simulink model "Sim_3_observer_performance_no_noise"  (R2019b)
settings: Solver=VariableStepAuto  StartTime=0.0  StopTime=sim_time  FixedStep=0.01  MaxStep=0.1  MinStep=0.0001  RelTol=0.01  AbsTol=0.01
values from neighbouring files (symbols this model uses):
  Controller_Data = struct('K_p', K_p, 'K_v', K_v, 'K_i', K_i, 'M', M,     'D', D, 'U_ref', U_ref, 'mu', mu)    [Sim_10_init.m]    (also in Sim_11_init.m; Sim_12_init.m; Sim_3_4_and_5_init.m; Sim_7_8_userdef_init.m)
  D = [ 0.66  0    0 ... (first row only)    [Sim_10_init.m]    (also in Sim_11_init.m; Sim_12_init.m; Sim_3_4_and_5_init.m; Sim_7_8_userdef_init.m)
  K_p = 0.08*[1.1  0    0 ... (first row only)    [Sim_10_init.m]    (also in Sim_11_init.m; Sim_12_init.m; Sim_3_4_and_5_init.m; Sim_7_8_userdef_init.m)
  K_v = 1*[10   0       0 ... (first row only)    [Sim_10_init.m]    (also in Sim_11_init.m; Sim_12_init.m; Sim_3_4_and_5_init.m; Sim_7_8_userdef_init.m = 3*[10   0       0)
  LossOfSignalFalse = 1    [Sim_10_init.m]    (also in Sim_11_init.m; Sim_12_init.m; Sim_3_4_and_5_init.m; Sim_7_8_userdef_init.m)
  LossOfSignalTime = 10    [Sim_10_init.m]    (also in Sim_11_init.m; Sim_12_init.m; Sim_3_4_and_5_init.m = 30; Sim_7_8_userdef_init.m)
  LossOfSignalTrue = 0    [Sim_10_init.m]    (also in Sim_11_init.m; Sim_12_init.m; Sim_3_4_and_5_init.m; Sim_7_8_userdef_init.m)
  M = [ 16    0      0 ... (first row only)    [Sim_10_init.m]    (also in Sim_11_init.m; Sim_12_init.m; Sim_3_4_and_5_init.m; Sim_7_8_userdef_init.m)
  mu = 0.09    [Sim_10_init.m]    (also in Sim_11_init.m; Sim_12_init.m; Sim_3_4_and_5_init.m; Sim_7_8_userdef_init.m)
  Observergains = [L1, L2, L3]    [Sim_10_init.m]    (also in Sim_11_init.m; Sim_12_init.m; Sim_3_4_and_5_init.m; Sim_7_8_userdef_init.m)
  path_planner_data = [start_pos; end_pos; Radius; Center]    [Sim_10_init.m]    (also in Sim_11_init.m; Sim_12_init.m; Sim_3_4_and_5_init.m; Sim_7_8_userdef_init.m)
  pathparameter = 0    [Sim_10_init.m]    (also in Sim_11_init.m = 1; Sim_12_init.m; Sim_3_4_and_5_init.m = 1; Sim_7_8_userdef_init.m = 1)
  RegainOfSignalFalse = 0    [Sim_10_init.m]    (also in Sim_11_init.m; Sim_12_init.m; Sim_3_4_and_5_init.m; Sim_7_8_userdef_init.m)
  RegainOfSignalTime = 30    [Sim_10_init.m]    (also in Sim_11_init.m; Sim_12_init.m; Sim_3_4_and_5_init.m = 50; Sim_7_8_userdef_init.m)
  RegainOfSignalTrue = 1    [Sim_10_init.m]    (also in Sim_11_init.m; Sim_12_init.m; Sim_3_4_and_5_init.m; Sim_7_8_userdef_init.m)
  start_pos = [10; 20; pi/2 ]    [Sim_10_init.m]    (also in Sim_11_init.m = [0; 0; 0 ]; Sim_12_init.m = [0; 0; 0 ]; Sim_3_4_and_5_init.m = [0; 0; 0 ]; Sim_7_init.m = [0; 0; 0 ])
undefined symbols (not defined in the file or in its folder): tsamp, WP
(part 2 of 3)

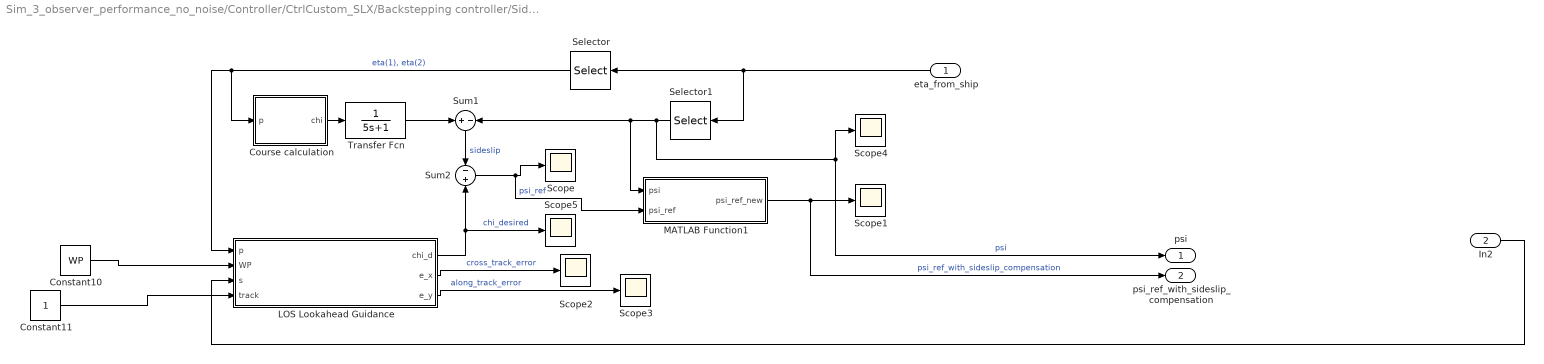
== system Sim_3_observer_performance_no_noise/Controller/CtrlCustom_SLX/Backstepping controller/Sideslip compensation  ==
  eta_from_ship : Inport
  In2 : Inport  Port=2
  Constant10 : Constant  Value=WP
  Constant11 : Constant
  Course calculation : MATLAB Function  TreatAsAtomicUnit=on  SystemSampleTime=tsamp
  LOS Lookahead Guidance : MATLAB Function  TreatAsAtomicUnit=on  SystemSampleTime=tsamp
  MATLAB Function1 : MATLAB Function  TreatAsAtomicUnit=on
  Scope{,1..5} (6 alike) : Scope
  Selector : Selector  InputPortWidth=3  IndexOptions=Index vector (dialog)  Indices=[1 2]  OutputSizes=1
  Selector1 : Selector  InputPortWidth=3  IndexOptions=Index vector (dialog)  Indices=[3]  OutputSizes=1
  Sum1 : Sum  Inputs=+-
  Sum2 : Sum  Inputs=-+
  Transfer Fcn : TransferFcn  Denominator=[5 1]
  psi : Outport
  psi_ref_with_sideslip_compensation : Outport  Port=2
  wires:
  Constant11/1 -> LOS Lookahead Guidance/4(track)
  Selector/1 -> LOS Lookahead Guidance/1(p), Course calculation/1(p)  "eta(1), eta(2)"
  eta_from_ship/1 -> Selector1/1, Selector/1
  Course calculation/1(chi) -> Transfer Fcn/1
  Sum1/1 -> Sum2/1  "sideslip"
  LOS Lookahead Guidance/1(chi_d) -> Sum2/2, Scope5/1  "chi_desired"
  Sum2/1 -> MATLAB Function1/2(psi_ref), Scope/1  "psi_ref"
  Transfer Fcn/1 -> Sum1/1
  LOS Lookahead Guidance/3(e_y) -> Scope3/1  "along_track_error"
  Selector1/1 -> psi/1, Scope4/1, Sum1/2, MATLAB Function1/1(psi)  "psi"
  In2/1 -> LOS Lookahead Guidance/3(s)
  Constant10/1 -> LOS Lookahead Guidance/2(WP)
  LOS Lookahead Guidance/2(e_x) -> Scope2/1  "cross_track_error"
  MATLAB Function1/1(psi_ref_new) -> psi_ref_with_sideslip_compensation/1, Scope1/1  "psi_ref_with_sideslip_compensation"

== system Sim_3_observer_performance_no_noise/Controller/DP_Ctrl/Backstepping controller/1//|p_d'| ==
  s : Inport
  switch : Inport  Port=2
  Elipse : MATLAB Function  TreatAsAtomicUnit=on
  Straight line : MATLAB Function  TreatAsAtomicUnit=on
  Switch : Switch  Criteria=u2 > Threshold
  1/|p_d'| : Outport
  wires:
  s/1 -> Elipse/1(s)
  Elipse/1(y) -> Switch/3
  Switch/1 -> 1/|p_d'|/1
  Straight line/1(y) -> Switch/1
  switch/1 -> Switch/2

== system Sim_3_observer_performance_no_noise/Controller/DP_Ctrl/Backstepping controller/Final_Tau_Computation ==
  alpha_1 : Inport
  alpha_1_dot : Inport  Port=2
  nu_hat : Inport  Port=3
  Gain : Gain  Gain=K_v  Multiplication=Matrix(K*u)
  Gain1 : Gain  Gain=M  Multiplication=Matrix(K*u)
  Gain2 : Gain  Gain=D  Multiplication=Matrix(K*u)
  Sum : Sum  Inputs=-+|
  Sum1 : Sum  Inputs=++-
  Tau : Outport
  wires:
  nu_hat/1 -> Sum/2
  alpha_1/1 -> Gain2/1, Sum/1
  Sum/1 -> Gain/1  "z_2"
  Sum1/1 -> Tau/1
  Gain/1 -> Sum1/3
  alpha_1_dot/1 -> Gain1/1
  Gain1/1 -> Sum1/1
  Gain2/1 -> Sum1/2

== system Sim_3_observer_performance_no_noise/Controller/DP_Ctrl/Backstepping controller/U_s(s) ==
  s : Inport
  switch : Inport  Port=2
  Eliptical : MATLAB Function  TreatAsAtomicUnit=on
  Straight line : MATLAB Function  TreatAsAtomicUnit=on
  Switch : Switch  Criteria=u2 > Threshold
  U_s : Outport
  wires:
  Straight line/1(y) -> Switch/1
  Switch/1 -> U_s/1
  Eliptical/1(y) -> Switch/3
  s/1 -> Eliptical/1(s)
  switch/1 -> Switch/2

== system Sim_3_observer_performance_no_noise/Controller/DP_Ctrl/Backstepping controller/U_s(s)' ==
  s : Inport
  "switch " : Inport  Port=2
  Constant : Constant  Value=0
  Elliptical : MATLAB Function  TreatAsAtomicUnit=on
  Switch : Switch  Criteria=u2 > Threshold
  U_s' : Outport
  wires:
  s/1 -> Elliptical/1(s)
  Elliptical/1(U_sf) -> Switch/3
  Switch/1 -> U_s'/1
  Constant/1 -> Switch/1
  "switch "/1 -> Switch/2

== system Sim_3_observer_performance_no_noise/Controller/DP_Ctrl/Backstepping controller/alpha_1, z_1 - explicit  ==
  eta : Inport
  eta_d(s) : Inport  Port=2
  eta_d(s)' : Inport  Port=3
  U_s : Inport  Port=4
  Gain : Gain  Gain=-K_p
  Product : Product
  Product1 : Product  Inputs=3
  Rotation Matrix : MATLAB Function  TreatAsAtomicUnit=on
  Selector : Selector  InputPortWidth=3  IndexOptions=Index vector (dialog)  Indices=[3]  OutputSizes=1
  Sum : Sum  Inputs=|+-
  Sum1 : Sum  Inputs=|++
  Transpose : Math  Operator=transpose  SignedPower=off  SaturateOnIntegerOverflow=on
  alpha_1 : Outport
  z_1 : Outport  Port=2
  wires:
  eta/1 -> Sum/1, Selector/1
  Selector/1 -> Rotation Matrix/1(psi)
  eta_d(s)/1 -> Sum/2
  Sum/1 -> Product/2
  Rotation Matrix/1(R_psi) -> Transpose/1
  Product/1 -> Gain/1, z_1/1
  Gain/1 -> Sum1/1
  Sum1/1 -> alpha_1/1
  Transpose/1 -> Product1/1, Product/1
  Product1/1 -> Sum1/2
  eta_d(s)'/1 -> Product1/2
  U_s/1 -> Product1/3

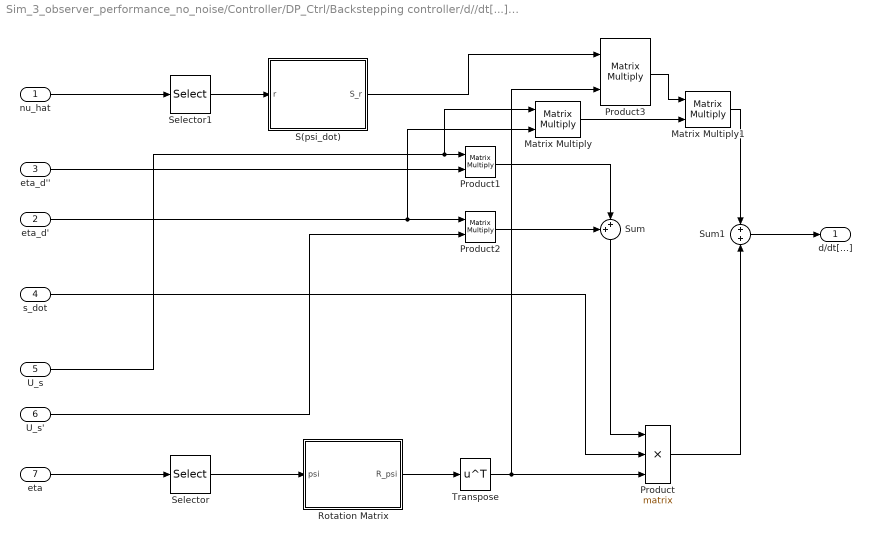
== system Sim_3_observer_performance_no_noise/Controller/DP_Ctrl/Backstepping controller/d//dt[...] calculation subsystem ==
  nu_hat : Inport
  eta_d' : Inport  Port=2
  eta_d'' : Inport  Port=3
  s_dot : Inport  Port=4
  U_s : Inport  Port=5
  "U_s' " : Inport  Port=6
  "eta " : Inport  Port=7
  Matrix Multiply : Product  Multiplication=Matrix(*)
  Matrix Multiply1 : Product  Multiplication=Matrix(*)
  Product : Product  Inputs=3  Multiplication=Matrix(*)
  Product1 : Product  Multiplication=Matrix(*)
  Product2 : Product  Multiplication=Matrix(*)
  Product3 : Product  Multiplication=Matrix(*)
  Rotation Matrix : MATLAB Function  TreatAsAtomicUnit=on
  S(psi_dot) : MATLAB Function  TreatAsAtomicUnit=on
  Selector : Selector  InputPortWidth=3  IndexOptions=Index vector (dialog)  Indices=[3]  OutputSizes=1
  Selector1 : Selector  InputPortWidth=3  IndexOptions=Index vector (dialog)  Indices=[3]  OutputSizes=1
  Sum : Sum  Inputs=++|
  Sum1 : Sum
  Transpose : Math  Operator=transpose  SignedPower=off  SaturateOnIntegerOverflow=on
  d/dt[...] : Outport
  wires:
  "eta "/1 -> Selector/1
  Selector/1 -> Rotation Matrix/1(psi)
  Rotation Matrix/1(R_psi) -> Transpose/1
  Transpose/1 -> Product3/2, Product/3
  s_dot/1 -> Product/2
  eta_d''/1 -> Product1/2
  U_s/1 -> Matrix Multiply/1, Product1/1
  Sum/1 -> Product/1
  Product1/1 -> Sum/2
  eta_d'/1 -> Matrix Multiply/2, Product2/1
  "U_s' "/1 -> Product2/2
  Product2/1 -> Sum/1
  nu_hat/1 -> Selector1/1
  Selector1/1 -> S(psi_dot)/1("r ")
  S(psi_dot)/1(S_r) -> Product3/1
  Product/1 -> Sum1/2
  Sum1/1 -> d/dt[...]/1
  Matrix Multiply/1 -> Matrix Multiply1/2
  Product3/1 -> Matrix Multiply1/1
  Matrix Multiply1/1 -> Sum1/1

== system Sim_3_observer_performance_no_noise/Controller/DP_Ctrl/Backstepping controller/eta_d''(s) ==
  s : Inport
  switch : Inport  Port=2
  Constant : Constant  Value=[0 0 0]'
  Elliptical : MATLAB Function  TreatAsAtomicUnit=on
  Switch : Switch  Criteria=u2 > Threshold
  "eta_d''(s) " : Outport
  wires:
  s/1 -> Elliptical/1(s)
  Elliptical/1(y) -> Switch/3
  Switch/1 -> "eta_d''(s) "/1
  Constant/1 -> Switch/1
  switch/1 -> Switch/2

== system Sim_3_observer_performance_no_noise/Controller/DP_Ctrl/Backstepping controller/eta_d'(s) ==
  s : Inport
  switch : Inport  Port=2
  Elliptical : MATLAB Function  TreatAsAtomicUnit=on
  Straight line : MATLAB Function  TreatAsAtomicUnit=on
  Switch : Switch  Criteria=u2 > Threshold
  Out1 : Outport
  wires:
  s/1 -> Elliptical/1(s)
  Elliptical/1(y) -> Switch/3
  Switch/1 -> Out1/1
  Straight line/1(y) -> Switch/1
  switch/1 -> Switch/2

== system Sim_3_observer_performance_no_noise/Controller/DP_Ctrl/Backstepping controller/eta_d(s) ==
  s : Inport
  switch : Inport  Port=2
  Eliptical path : MATLAB Function  TreatAsAtomicUnit=on
  Straight line : MATLAB Function  TreatAsAtomicUnit=on
  Switch : Switch  Criteria=u2 > Threshold
  "eta_d''(s) " : Outport
  wires:
  s/1 -> Straight line/1(s), Eliptical path/1(s)
  Eliptical path/1(y) -> Switch/3
  Switch/1 -> "eta_d''(s) "/1
  Straight line/1(y) -> Switch/1
  switch/1 -> Switch/2

== system Sim_3_observer_performance_no_noise/Controller/DP_Ctrl/Backstepping controller/z_1_dot subsystem  ==
  eta_d : Inport
  eta_d' : Inport  Port=2
  eta : Inport  Port=3
  s_dot : Inport  Port=4
  nu_hat : Inport  Port=5
  Product : Product  Inputs=3  Multiplication=Matrix(*)
  Product1 : Product  Inputs=3  Multiplication=Matrix(*)
  Rotation Matrix : MATLAB Function  TreatAsAtomicUnit=on
  S(psi_dot) : MATLAB Function  TreatAsAtomicUnit=on
  Selector : Selector  InputPortWidth=3  IndexOptions=Index vector (dialog)  Indices=[3]  OutputSizes=1
  Selector1 : Selector  InputPortWidth=3  IndexOptions=Index vector (dialog)  Indices=[3]  OutputSizes=1
  Sum : Sum  Inputs=-+|
  Sum1 : Sum  Inputs=+++
  Transpose : Math  Operator=transpose  SignedPower=off  SaturateOnIntegerOverflow=on
  Transpose1 : Math  Operator=transpose  SignedPower=off  SaturateOnIntegerOverflow=on
  Transpose3 : Math  Operator=transpose  SignedPower=off  SaturateOnIntegerOverflow=on
  z_1_dot : Outport
  wires:
  nu_hat/1 -> Sum1/3, Selector/1
  Selector/1 -> S(psi_dot)/1("r ")
  eta/1 -> Selector1/1, Sum/2
  eta_d/1 -> Sum/1
  Selector1/1 -> Rotation Matrix/1(psi)
  Rotation Matrix/1(R_psi) -> Transpose1/1
  Sum/1 -> Product/1
  S(psi_dot)/1(S_r) -> Transpose/1
  Transpose/1 -> Product/3
  Sum1/1 -> Transpose3/1
  Product/1 -> Sum1/2
  s_dot/1 -> Product1/2
  eta_d'/1 -> Product1/1
  Product1/1 -> Sum1/1
  Transpose1/1 -> Product/2, Product1/3
  Transpose3/1 -> z_1_dot/1

== system Sim_3_observer_performance_no_noise/Controller/DP_Ctrl/Thrust Allocation /u ==
  In1 : Inport
  Constant : Constant  Value=0.3
  Constant1 : Constant  Value=0.3
  Demux1 : Demux  Outputs=5
  Mux : Mux  Inputs=7
  Saturation1 : Saturate  UpperLimit=1  LowerLimit=0
  Saturation11 : Saturate  UpperLimit=1  LowerLimit=0
  Out1 : Outport  VectorParamsAs1DForOutWhenUnconnected=off
  wires:
  In1/1 -> Demux1/1
  Demux1/1 -> Mux/1  "u_BT"
  Demux1/2 -> Saturation11/1  "u_VSP1"
  Demux1/3 -> Saturation1/1  "u_VSP2"
  Demux1/4 -> Mux/4  "alpha_VSP1"
  Demux1/5 -> Mux/5  "alpha_VSP2"
  Constant/1 -> Mux/6  "omega_VSP1"
  Constant1/1 -> Mux/7  "omega_VSP2"
  Mux/1 -> Out1/1
  Saturation11/1 -> Mux/2
  Saturation1/1 -> Mux/3

== matlab function Sim_3_observer_performance_no_noise/Simulator CSE1/EquationsOfMotion (Fossen Model)/kinematics ==
  data: nu input size=3; eta_dot output size=3; eta input size=3
function eta_dot = CSE1_eta_dot(nu,eta)

psi = eta(3);

J = [cos(psi) -sin(psi) 0
     sin(psi) cos(psi)  0
     0        0         1];

eta_dot = J*nu;

== matlab function Sim_3_observer_performance_no_noise/Simulator CSE1/EquationsOfMotion (Fossen Model)/kinetics ==
  data: tau input; nu_dot output; nu input
function nu_dot = CSE1_nu_dot(tau,nu)

u   = nu(1);
v   = nu(2);
r   = nu(3);

tau = [tau(1);tau(2);tau(3)];
%% MATRICES 
%changed m from 14.79 to 14.11

m    = 14.11;   I_z  =  1.7600;   x_g = 0.0375;       % x_g  =  0.0460; % Table B.1

%% Added mass
%changed Y_vd from -1.0 to -10.0
X_ud  =     -2.0;											% Table B.1
					Y_vd =      -10.0;	N_vd =    -0.0;		% Table B.1
					Y_rd =      -0.0;	N_rd =    -1.0;		% Table B.1

%% Total mass matrix
m_11 = m-X_ud;
m_22 = m-Y_vd;
m_23 = m*x_g-Y_rd;
m_32 = m*x_g-N_vd; % noted as Y_rd in handbook, but same value
m_33 = I_z-N_rd;

M    = [m_11 0    0
        0    m_22 m_23
        0    m_32 m_33];
	
%% Damping coefficients
% Comments at the end of the lines indicate the old values used.
X_u		= -0.6555;		X_v		= 0;
X_uu 	= 0.3545;		X_vv	= -2.443;
X_uuu 	= -3.787;		X_vvv	= 0;

						Y_v		= -1.33; 			Y_r		= -7.250; % Y_r
						Y_vv	= -2.776;			Y_rr	= -3.450; % Y_rr
						Y_vvv	= -64.91;			Y_rrr	= 0;
						
						Y_rv	= -0.805;			Y_vr	= -0.845; % Y_rv, Y_vr

						N_v		= 0;				N_r		= -1.900; % N_r
						N_vv	= -0.2088;			N_rr	= -0.750; % N_rr
						N_vvv	= 0;				N_rrr	= 0;
						
						N_rv	= 0.130;			N_vr	= 0.080; % N_rv, N_vr

%% Correolis matrix
c_13 = -(m-Y_vd)*v-(m*x_g-Y_rd)*r;
c_23 = (m-X_ud)*u;
C    = [0     0     c_13
        0     0     c_23
        -c_13 -c_23 0   ];

%% Assembly of the damping matrix
%should be abs(u), abs(v) some places, only positive values? 

d_11 = -X_u - X_uu*u - X_uuu*u^2;
d_22 = -Y_v - Y_vv*v - Y_vvv*v^2 - Y_rv*abs(r);
d_33 = -N_r - N_rr*abs(r) - N_rrr*r^2 - N_vr*abs(v); % using abs(r)

d_12 = -X_v - X_vv*v - X_vvv*v^2;
d_23 = -Y_r - Y_rr*abs(r) - Y_rrr*r^2 - Y_vr*abs(v);
d_32 = -N_v - N_vv*v - N_vvv*v^2 - N_rv*abs(r);

%D    = [d_11 d_12 0      vet ikke hvorfor d_12 er her
%        0    d_22 d_23
%        0    d_32 d_33];
D    = [d_11 0 0
        0    d_22 d_23
        0    d_32 d_33];


%% CALCULATION
nu_dot = M\(tau-(C+D)*nu);

== matlab function Sim_3_observer_performance_no_noise/Simulator CSE1/EquationsOfMotion (Fossen Model)/MATLAB Function ==
  data: psi input; BodyVector output; NedVector input
function BodyVector = fcn(psi,NedVector)
R=[cos(psi) sin(psi) 0; -sin(psi) cos(psi) 0;0 0 1];
BodyVector=R*NedVector;
end

== matlab function Sim_3_observer_performance_no_noise/Wrap2QualisysOutput /Wrap2psi ==
  data: u input; yQualisus output
function yQualisus = fcn(u)
y=sin(u);
x=cos(u);
yQualisus=atan2(y,x);
end

== matlab function Sim_3_observer_performance_no_noise/WrapPsiTo[-pi,pi]1/Wrap2psi1 ==
  data: u input; yQualisus output
function yQualisus = fcn(u)
y=sin(u);
x=cos(u);
yQualisus=atan2(y,x);
end

== matlab function Sim_3_observer_performance_no_noise/WrapPsiTo[-pi,pi]2/Wrap2psi1 ==
  data: u input; yQualisus output
function yQualisus = fcn(u)
y=sin(u);
x=cos(u);
yQualisus=atan2(y,x);
end

== matlab function Sim_3_observer_performance_no_noise/Controller/CtrlCustom_SLX/beta  ==
  data: u_star input; u_cmd output; alpha input; alpha_cmd output
function [ u_cmd , alpha_cmd ] = beta ( u_star , alpha )

for i=1:2
    if u_star(i) < 0
        u_star(i) = abs(u_star(i));
        alpha(i) = alpha(i) - pi;
        if alpha(i) <= -pi
            alpha(i) = alpha(i) + 2*pi ;
        end
    end
    
    if u_star(i) > 1 
        u_star(i) = 1;
    end
end

u_cmd = u_star;
alpha_cmd = alpha;

end

== matlab function Sim_3_observer_performance_no_noise/Controller/Switch_function ==
  data: Cross_1 input; switch_signal output; Square_2 input; Circle_3 input; Triangle_4 input; temp input
%% Function that takes in impulse button sigals [0,1] and sends out a 
% different signal depentent pn which button has been pressed

function switch_signal = fcn(Cross_1,Square_2,Circle_3,Triangle_4,temp)
%#codegen
persistent signal;

signal = temp;

if Cross_1 ~= 0
    signal = 1;
end

if Square_2 ~= 0
    signal = 2;
end

if Circle_3 ~= 0
    signal = 3;
end
    
if Triangle_4 ~= 0
    signal = 4; 
end

switch_signal = signal;

== matlab function Sim_3_observer_performance_no_noise/Controller/Sixais Sim ==
  data: Selector input; Out output
%% Function that takes in impulse button sigals [0,1] and sends out a 
% different signal depentent pn which button has been pressed

function Out = fcn(Selector)
%#codegen
if Selector==1
    Out=[1 0 0 0];
elseif Selector==2
        Out=[0 1 0 0];
elseif Selector==4
        Out=[0 0 0 1];
else 
        Out=[0 0 1 0];

end

== matlab function Sim_3_observer_performance_no_noise/Controller/DP_Ctrl/Thrust Allocation /beta  ==
  data: u_star input; u_cmd output; alpha input; alpha_cmd output
function [ u_cmd , alpha_cmd ] = beta ( u_star , alpha )

for i=1:2
    if u_star(i) < 0
        u_star(i) = abs(u_star(i));
        alpha(i) = alpha(i) - pi;
        if alpha(i) <= -pi
            alpha(i) = alpha(i) + 2*pi ;
        end
    end
    
    if u_star(i) > 1 
        u_star(i) = 1;
    end
end

u_cmd = u_star;
alpha_cmd = alpha;

end

== matlab function Sim_3_observer_performance_no_noise/Controller/CtrlCustom_SLX/beta 1 ==
  data: u_star input; u_cmd output size=3; alpha input; alpha_cmd output size=2
function [ u_cmd , alpha_cmd ] = beta ( u_star , alpha )

for i=1:2
    if u_star(i) < 0
        u_star(i) = abs(u_star(i));
        alpha(i) = alpha(i) - pi;
        if alpha(i) < -pi
            alpha(i) = alpha(i) + 2*pi ;
        end
    end
%     alpha
%Saturate VSP to give maximum 100% thrust    
    if u_star(i) > 1 
        u_star(i) = 1;
    end
end

%Saturate bow thruster to a maximum of 1 (100% thrust)
if(u_star(3) > 1)
    u_star(3) = 1;
elseif u_star(3) <-1
    u_star(3) = -1;
end

u_cmd = u_star;
alpha_cmd = alpha;

end

== matlab function Sim_3_observer_performance_no_noise/Simulator CSE1/B Command to force mapping/Bow thruster ==
  data: u_BT input; F_y output; nu input
function F_y = fcn(u_BT,nu)
%#codegen
u = nu(1);
% Thruster characteristics
if u_BT >0
    u_BT=u_BT+ 0.059;
    a =        -548;
    b =       0.193;
    c =       548.2;
    d =      0.1992;
    y0 = -(a*exp(b*-u_BT) + c*exp(d*-u_BT));
elseif u_BT < 0
    u_BT=u_BT- 0.059;
    a =        -548;
    b =       0.193;
    c =       548.2;
    d =      0.1992;
    y0 = a*exp(b*u_BT) + c*exp(d*u_BT);
else
    y0 = 0;
end
% Thruster losses due to forward speed
a0 =      0.7561;
a1 =      0.3075;
b1 =      -10.22;
c1 =       2.947;
F_y = y0*(a0 + a1*atan(b1*u +c1))/1.1385;
F_y=F_y*2.62/2.7629;


%2019 changes- Some add-hock changes, because it did not make sense previously.

== matlab function Sim_3_observer_performance_no_noise/Simulator CSE1/B Command to force mapping/VSP ==
  data: alpha input; F_x output; u_VSP input; F_y output
function [ F_x , F_y ] = fcn(alpha,u_VSP)
%#codegen
% Calculating the force in x-direction
a1 =       1.107  ;
b1 =       1.001  ;
c1 =       1.564  ;
a2 =      0.3471 ;
b2 =      0.1397 ;
c2 =      -1.599  ;
a3 =      0.1558 ;
b3 =       1.993  ;
c3 =       1.886  ;
a4 =      0.1599 ;
b4 =       0.218  ;
c4 =       1.513  ;
a5 =     0.08237 ;
b5 =       2.986  ;
c5 =      -1.601  ;
a6 =     0.04641 ;
b6 =       3.964  ;
c6 =       1.738  ;
F_x =   u_VSP*( a1*sin(b1*alpha+c1) + ...
                a2*sin(b2*alpha+c2) + ...
                a3*sin(b3*alpha+c3) + ...
                a4*sin(b4*alpha+c4) + ...
                a5*sin(b5*alpha+c5) + ...
                a6*sin(b6*alpha+c6) );
% Calculating the force in y-direction
a1 =      0.7936 ;
b1 =       1.001  ;
c1 =     0.01605;
a2 =      0.2112 ;
b2 =       1.997  ;
c2 =     0.03229;
a3 =     0.07608;
b3 =       2.991  ;
c3 =       2.986  ;
a4 =     0.04817;
b4 =       3.999  ;
c4 =     -0.8668 ;
a5 =     0.01757;
b5 =       4.904  ;
c5 =      -2.622 ;
a6 =    -0.02089;
b6 =       5.068  ;
c6 =      0.2548 ;
F_y =   u_VSP*( a1*sin(b1*alpha+c1) + ...
                a2*sin(b2*alpha+c2) + ...
                a3*sin(b3*alpha+c3) + ...
                a4*sin(b4*alpha+c4) + ...
                a5*sin(b5*alpha+c5) + ...
                a6*sin(b6*alpha+c6));

== matlab function Sim_3_observer_performance_no_noise/Simulator CSE1/B Command to force mapping/VSP1 ==
  data: alpha input; F_x output; u_VSP input; F_y output
function [ F_x , F_y ] = fcn(alpha,u_VSP)
%#codegen
% Calculating the force in x-direction
a1 =       1.107  ;
b1 =       1.001  ;
c1 =       1.564  ;
a2 =      0.3471 ;
b2 =      0.1397 ;
c2 =      -1.599  ;
a3 =      0.1558 ;
b3 =       1.993  ;
c3 =       1.886  ;
a4 =      0.1599 ;
b4 =       0.218  ;
c4 =       1.513  ;
a5 =     0.08237 ;
b5 =       2.986  ;
c5 =      -1.601  ;
a6 =     0.04641 ;
b6 =       3.964  ;
c6 =       1.738  ;
F_x =   u_VSP*( a1*sin(b1*alpha+c1) + ...
                a2*sin(b2*alpha+c2) + ...
                a3*sin(b3*alpha+c3) + ...
                a4*sin(b4*alpha+c4) + ...
                a5*sin(b5*alpha+c5) + ...
                a6*sin(b6*alpha+c6) );
% Calculating the force in y-direction
a1 =      0.7936 ;
b1 =       1.001  ;
c1 =     0.01605;
a2 =      0.2112 ;
b2 =       1.997  ;
c2 =     0.03229;
a3 =     0.07608;
b3 =       2.991  ;
c3 =       2.986  ;
a4 =     0.04817;
b4 =       3.999  ;
c4 =     -0.8668 ;
a5 =     0.01757;
b5 =       4.904  ;
c5 =      -2.622 ;
a6 =    -0.02089;
b6 =       5.068  ;
c6 =      0.2548 ;
F_y =   u_VSP*( a1*sin(b1*alpha+c1) + ...
                a2*sin(b2*alpha+c2) + ...
                a3*sin(b3*alpha+c3) + ...
                a4*sin(b4*alpha+c4) + ...
                a5*sin(b5*alpha+c5) + ...
                a6*sin(b6*alpha+c6));

== matlab function Sim_3_observer_performance_no_noise/Controller/CtrlCustom_SLX/fixed azimuth thrust allocation  ==
  data: tau_ref input; u_cmd output; alpha input; alpha_cmd output
function [ u_cmd , alpha_cmd ] = fcn(tau_ref , alpha)

k1 = 1.030; k2 = 1.030; k3 = 2.629;
k = [k1;k2;k3];
K = diag(k);    %Thrust coefficient matrix

Lx = -0.4574; Ly = 0.055; L_BT = 0.3875;  %Thruster cooridinates

B_alpha = [                      cos(alpha(1))                     ,                   cos(alpha(2))                        ,   0 ; 
                                         sin(alpha(1))                     ,                    sin(alpha(2))                         ,   1 ;
                     - Ly * cos(alpha(1)) + Lx * sin(alpha(1)) , Ly * cos(alpha(2)) + Lx * sin(alpha(2)) , L_BT ];

u_cmd = pinv(B_alpha*K) * tau_ref;
alpha_cmd = alpha;

end

== matlab function Sim_3_observer_performance_no_noise/Controller/CtrlCustom_SLX/varying azimuth thrust allocation ==
  data: tau_ref input; u_cmd output; alpha_cmd output
function [ u_cmd , alpha_cmd ] = fcn(tau_ref)

k1 = 1.030; k2 = 1.030; k3 = 2.629;
k = [k1;k1;k2;k2;k3];
K = diag(k);    %Thrust coefficient matrix

Lx = -0.4574; Ly = 0.055; L_BT = 0.3875;  %Thruster cooridinates

B_alpha = [ 1, 0, 1, 0, 0 ;
            0, 1, 0, 1, 1 ;
           -Ly, Lx, Ly, Lx, L_BT];
            
u_star = pinv( B_alpha * K ) * tau_ref ;

u_cmd = zeros(3,1);
alpha_cmd = zeros(2,1);

u_cmd(1) = sqrt(u_star(1)^2 + u_star(2)^2) ;
u_cmd(2) = sqrt(u_star(3)^2 + u_star(4)^2) ;
u_cmd(3) = u_star(5) ;

%%Returns values in [-pi/2, pi/2]
% alpha_cmd(1) = atan(u_star(2)/u_star(1));
% alpha_cmd(2) = atan(u_star(4)/u_star(3));

% Returns angles in  [-pi, pi]
alpha_cmd(1) = atan2(u_star(2),u_star(1));
alpha_cmd(2) = atan2(u_star(4),u_star(3));
end

== matlab function Sim_3_observer_performance_no_noise/Controller/Subsystem/Rotation Matrix ==
  data: psi input; R_psi output
function R_psi = fcn(psi)
R_psi = [ cos(psi)  -sin(psi)   0  ;
                sin(psi)    cos(psi)  0  ; 
                    0              0         1  ] ;
end

== matlab function Sim_3_observer_performance_no_noise/Controller/Subsystem/Transpose Rotation Matrix ==
  data: psi input; R_psi_trans output
function R_psi_trans = fcn(psi)
R_psi = [ cos(psi)  -sin(psi)   0  ;
                sin(psi)    cos(psi)  0  ; 
                    0              0         1  ] ;
                
R_psi_trans = transpose(R_psi);
end

== matlab function Sim_3_observer_performance_no_noise/Controller/Subsystem/S(psi_dot) ==
  data: r input; S_r output
function S_r = fcn(r)
S_r = [ 0  -r   0  ;
         r  0   0   ; 
         0  0   1  ] ;
end

== matlab function Sim_3_observer_performance_no_noise/Controller/Subsystem/z_1_dot subsystem /S(psi_dot) ==
  data: r input; S_r output
function S_r = fcn(r)
S_r = [ 0  -r   0  ;
         r  0   0   ; 
         0  0   1  ] ;
end

== matlab function Sim_3_observer_performance_no_noise/Controller/Subsystem/z_1_dot subsystem /Rotation Matrix ==
  data: psi input; R_psi output
function R_psi = fcn(psi)
R_psi = [ cos(psi)  -sin(psi)   0  ;
                sin(psi)    cos(psi)  0  ; 
                    0              0         1  ] ;
end

== matlab function Sim_3_observer_performance_no_noise/Controller/Subsystem/d//dt[...] calculation subsystem/Rotation Matrix ==
  data: psi input; R_psi output
function R_psi = fcn(psi)
R_psi = [ cos(psi)  -sin(psi)   0  ;
                sin(psi)    cos(psi)  0  ; 
                    0              0         1  ] ;
end

== matlab function Sim_3_observer_performance_no_noise/Controller/Subsystem/d//dt[...] calculation subsystem/S(psi_dot) ==
  data: r input; S_r output
function S_r = fcn(r)
S_r = [ 0  -r   0  ;
         r  0   0   ; 
         0  0   1  ] ;
end

== matlab function Sim_3_observer_performance_no_noise/Controller/Subsystem/alpha_1, z_1 - explicit /Rotation Matrix ==
  data: psi input; R_psi output
function R_psi = fcn(psi)
R_psi = [ cos(psi)  -sin(psi)   0  ;
                sin(psi)    cos(psi)  0  ; 
                    0              0         1  ] ;
end

== matlab function Sim_3_observer_performance_no_noise/Controller/Subsystem/U_s(s)/Straight line ==
  data: y output
function y = fcn()
x1 = 0;
y1 = 0;
x2 = 50;
y2= 50;
uref = 0.3;

y = uref/sqrt((x2-x1)^2+(y2-y1)^2);

== matlab function Sim_3_observer_performance_no_noise/Controller/Subsystem/U_s(s)/Eliptical ==
  data: s input; y output
function y = fcn(s)
Uref = 0.3;
rx = 1.5;
ry = 1;

y = Uref/sqrt((rx*2*pi*cos(2*pi*s))^2+(ry*2*pi*sin(2*pi*s))^2);

== matlab function Sim_3_observer_performance_no_noise/Controller/Subsystem/U_s(s)'/MATLAB Function ==
  data: s input; U_sf output
function U_sf = fcn(s)
Uref = 0.3;
rx = 1.5;
ry = 1;

xdf = (-rx*2*pi*sin(2*pi*s));
ydf = (ry*2*pi*cos(2*pi*s));
xdff = -rx(2*pi)^2*cos(2*pi*s);
ydff = -ry(2*pi)^2*sin(2*pi*s);

dhdxdf = -Uref*xdf/(xdf^2+ydf^2)^(3/2);
dhdydf = -Uref*ydf/((xdf^2+ydf^2)^(3/2));

U_sf = dhdxf*xdff + dhdyf*ydff;

== matlab function Sim_3_observer_performance_no_noise/Controller/Subsystem/1//|p_d'|/Elipse ==
  data: y output; s input
function y = fcn(s)
xdf = (-rx*2*pi*sin(2*pi*s));
ydf = (ry*2*pi*cos(2*pi*s));
y = 1/sqrt(xdf^2+ydf^2);

== matlab function Sim_3_observer_performance_no_noise/Controller/Subsystem/1//|p_d'|/Straight line ==
  data: y output
function y = fcn()
x1 = 0;
y1 = 0;
x2 = 50;
y2= 50;


y = 1/sqrt((x2-x1)^2+(y2-y1)^2);

== matlab function Sim_3_observer_performance_no_noise/Controller/Subsystem/eta_d'(s)/MATLAB Function ==
  data: s input; y output
function y = fcn(s)

xdf = (-rx*2*pi*sin(2*pi*s));
ydf = (ry*2*pi*cos(2*pi*s));
xdff = -rx(2*pi)^2*cos(2*pi*s);
ydff = -ry(2*pi)^2*sin(2*pi*s);
dfdydf =  xdf/(ydf^2+xdf^2);
dfdxdf = -ydf/(ydf^2+xdf^2);

psidf =dfdxdf*xdff+dfdydf*ydff; 
y = [xdf,ydf,psidf]';

== matlab function Sim_3_observer_performance_no_noise/Controller/Subsystem/eta_d'(s)/MATLAB Function1 ==
  data: y output
function y = fcn()
x1 = 0;
y1 = 0;
x2 = 50;
y2= 50;
y = [x2-x1, y2-y1, 0]';

== matlab function Sim_3_observer_performance_no_noise/Controller/Subsystem/eta_d''(s)/MATLAB Function ==
  data: s input; y output
function y = fcn(s)
rx = 1.5;
ry = 0.5;


xdf = (-rx*2*pi*cos(2*pi*s));
ydf = (ry*2*pi*sin(2*pi*s));
xdff = -rx(2*pi)^2*cos(2*pi*s);
ydff = -ry(2*pi)^2*sin(2*pi*s);
xdff = rx(2*pi)^3*sin(2*pi*s);
ydff = -ry(2*pi)^3*cos(2*pi*s);

df_dydf =  xdf/(ydf^2+xdf^2);
df_dxdf = -ydf/(ydf^2+xdf^2);
ddf_dxddf = 2*xdf*ydf/(xdf^2+ydf^2)^2;
ddf_ddydf = -2*xdf*ydf/(xdf^2+ydf^2)^2;
ddf_dxdfdydf = (ydf^2-xdf^2)/(ydf^2+cdf^2)^2;

psidff =ddf_dxddf*xdff^2+ddf_ddydf*ydff^2+2*ddf_dxdfdydf*xdff*ydff+df_dxdf*xdfff+df_dydf*ydfff; 
y = [xdff,ydff,psidff]';

== matlab function Sim_3_observer_performance_no_noise/Controller/Subsystem/eta_d(s)/Eliptical path ==
  data: s input; y output
function y = fcn(s)
rx = 1.5;
ry = 0.5;
Cx = 0;
Cy = 0;

xdf = (-rx*2*pi*sin(2*pi*s));
ydf = (ry*2*pi*cos(2*pi*s));

y = [Cx+rx*cos(2*pi*s),Cy+ry*sin(2*pi*s),atan2(ydf,xdf)]';

== matlab function Sim_3_observer_performance_no_noise/Controller/Subsystem/eta_d(s)/Straight line ==
  data: s input; y output
function y = fcn(s)
x1 = 0;
y1 = 0;
x2 = 50;
y2 = 50;


y = [s*x2+(1-s)*x1, s*y2+(1-s)*y1, atan2(y2-y1,x2-x1)];

== matlab function Sim_3_observer_performance_no_noise/Controller/DP_Ctrl/Backstepping controller/1//|p_d'|/Elipse ==
  data: y output; s input
function y = fcn(s)
xdf = (-rx*2*pi*sin(2*pi*s));
ydf = (ry*2*pi*cos(2*pi*s));
y = 1/sqrt(xdf^2+ydf^2);

== matlab function Sim_3_observer_performance_no_noise/Controller/DP_Ctrl/Backstepping controller/1//|p_d'|/Straight line ==
  data: y output
function y = fcn()
x1 = 0;
y1 = 0;
x2 = 50;
y2= 50;


y = 1/sqrt((x2-x1)^2+(y2-y1)^2);

== matlab function Sim_3_observer_performance_no_noise/Controller/DP_Ctrl/Backstepping controller/Rotation Matrix ==
  data: psi input; R_psi output
function R_psi = fcn(psi)
R_psi = [ cos(psi)  -sin(psi)   0  ;
                sin(psi)    cos(psi)  0  ; 
                    0              0         1  ] ;
end

== matlab function Sim_3_observer_performance_no_noise/Controller/DP_Ctrl/Backstepping controller/S(psi_dot) ==
  data: r input; S_r output
function S_r = fcn(r)
S_r = [ 0  -r   0  ;
         r  0   0   ; 
         0  0   1  ] ;
end

== matlab function Sim_3_observer_performance_no_noise/Controller/DP_Ctrl/Backstepping controller/Transpose Rotation Matrix ==
  data: psi input; R_psi_trans output
function R_psi_trans = fcn(psi)
R_psi = [ cos(psi)  -sin(psi)   0  ;
                sin(psi)    cos(psi)  0  ; 
                    0              0         1  ] ;
                
R_psi_trans = transpose(R_psi);
end

== matlab function Sim_3_observer_performance_no_noise/Controller/DP_Ctrl/Backstepping controller/U_s(s)/Eliptical ==
  data: s input; y output
function y = fcn(s)
Uref = 0.3;
rx = 1.5;
ry = 1;

y = Uref/sqrt((rx*2*pi*cos(2*pi*s))^2+(ry*2*pi*sin(init
2*pi*s))^2);

== matlab function Sim_3_observer_performance_no_noise/Controller/DP_Ctrl/Backstepping controller/U_s(s)/Straight line ==
  data: y output
function y = fcn()
x1 = 0;
y1 = 0;
x2 = 50;
y2= 50;
uref = 0.3;

y = uref/sqrt((x2-x1)^2+(y2-y1)^2);

== matlab function Sim_3_observer_performance_no_noise/Controller/DP_Ctrl/Backstepping controller/U_s(s)'/Elliptical ==
  data: s input; U_sf output
function U_sf = fcn(s)
Uref = 0.3;
rx = 1.5;
ry = 1;

xdf = (-rx*2*pi*sin(2*pi*s));
ydf = (ry*2*pi*cos(2*pi*s));
xdff = -rx*(2*pi)^2*cos(2*pi*s);
ydff = -ry*(2*pi)^2*sin(2*pi*s);

dhdxdf = -Uref*xdf/((xdf^2+ydf^2)^(3/2));
dhdydf = -Uref*ydf/((xdf^2+ydf^2)^(3/2));

U_sf = dhdxdf*xdff + dhdydf*ydff;

== matlab function Sim_3_observer_performance_no_noise/Controller/DP_Ctrl/Backstepping controller/alpha_1, z_1 - explicit /Rotation Matrix ==
  data: psi input; R_psi output
function R_psi = fcn(psi)
R_psi = [ cos(psi)  -sin(psi)   0  ;
                sin(psi)    cos(psi)  0  ; 
                    0              0         1  ] ;
end

== matlab function Sim_3_observer_performance_no_noise/Controller/DP_Ctrl/Backstepping controller/d//dt[...] calculation subsystem/Rotation Matrix ==
  data: psi input; R_psi output
function R_psi = fcn(psi)
R_psi = [ cos(psi)  -sin(psi)   0  ;
                sin(psi)    cos(psi)  0  ; 
                    0              0         1  ] ;
end

== matlab function Sim_3_observer_performance_no_noise/Controller/DP_Ctrl/Backstepping controller/d//dt[...] calculation subsystem/S(psi_dot) ==
  data: r input; S_r output
function S_r = fcn(r)
S_r = [ 0  -r   0  ;
         r  0   0   ; 
         0  0   1  ] ;
end

== matlab function Sim_3_observer_performance_no_noise/Controller/DP_Ctrl/Backstepping controller/eta_d''(s)/Elliptical ==
  data: s input; y output
function y = fcn(s)
rx = 1.5;
ry = 0.5;


xdf = (-rx*2*pi*cos(2*pi*s));
ydf = (ry*2*pi*sin(2*pi*s));
xdff = -rx*(2*pi)^2*cos(2*pi*s);
ydff = -ry*(2*pi)^2*sin(2*pi*s);
xdfff = rx*(2*pi)^3*sin(2*pi*s);
ydfff = -ry*(2*pi)^3*cos(2*pi*s);

df_dydf =  xdf/(ydf^2+xdf^2);
df_dxdf = -ydf/(ydf^2+xdf^2);
ddf_dxddf = 2*xdf*ydf/(xdf^2+ydf^2)^2;
ddf_ddydf = -2*xdf*ydf/(xdf^2+ydf^2)^2;
ddf_dxdfdydf = (ydf^2-xdf^2)/(ydf^2+xdf^2)^2;

psidff =ddf_dxddf*xdff^2+ddf_ddydf*ydff^2+2*ddf_dxdfdydf*xdff*ydff+df_dxdf*xdfff+df_dydf*ydfff; 
y = transpose([xdff,ydff,psidff]);

== matlab function Sim_3_observer_performance_no_noise/Controller/DP_Ctrl/Backstepping controller/eta_d'(s)/Elliptical ==
  data: s input; y output
function y = fcn(s)
rx = 1.5;
ry = 0.5;

xdf = (-rx*2*pi*sin(2*pi*s));
ydf = (ry*2*pi*cos(2*pi*s));
xdff = -rx*(2*pi)^2*cos(2*pi*s);
ydff = -ry*(2*pi)^2*sin(2*pi*s);
dfdydf =  xdf/(ydf^2+xdf^2);
dfdxdf = -ydf/(ydf^2+xdf^2);

psidf =dfdxdf*xdff+dfdydf*ydff; 
y = transpose([xdf,ydf,psidf]);

== matlab function Sim_3_observer_performance_no_noise/Controller/DP_Ctrl/Backstepping controller/eta_d'(s)/Straight line ==
  data: y output
function y = fcn()
x1 = 0;
y1 = 0;
x2 = 50;
y2= 50;
y = transpose([x2-x1, y2-y1, 0]);

== matlab function Sim_3_observer_performance_no_noise/Controller/DP_Ctrl/Backstepping controller/eta_d(s)/Eliptical path ==
  data: s input; y output
function y = fcn(s)
rx = 1.5;
ry = 0.5;
Cx = 0;
Cy = 0;

xdf = (-rx*2*pi*sin(2*pi*s));
ydf = (ry*2*pi*cos(2*pi*s));    

y = transpose([Cx+rx*cos(2*pi*s),Cy+ry*sin(2*pi*s),atan2(ydf,xdf)]);

== matlab function Sim_3_observer_performance_no_noise/Controller/DP_Ctrl/Backstepping controller/eta_d(s)/Straight line ==
  data: s input; y output
function y = fcn(s)
x1 = 0;
y1 = 0;
x2 = 50;
y2 = 50;


y = transpose([s*x2+(1-s)*x1, s*y2+(1-s)*y1, atan2(y2-y1,x2-x1)]);

== matlab function Sim_3_observer_performance_no_noise/Controller/DP_Ctrl/Backstepping controller/z_1_dot subsystem /Rotation Matrix ==
  data: psi input; R_psi output
function R_psi = fcn(psi)
R_psi = [ cos(psi)  -sin(psi)   0  ;
                sin(psi)    cos(psi)  0  ; 
                    0              0         1  ] ;
end

== matlab function Sim_3_observer_performance_no_noise/Controller/DP_Ctrl/Backstepping controller/z_1_dot subsystem /S(psi_dot) ==
  data: r input; S_r output
function S_r = fcn(r)
S_r = [ 0  -r   0  ;
         r  0   0   ; 
         0  0   1  ] ;
end

== matlab function Sim_3_observer_performance_no_noise/Controller/DP_Ctrl/Thrust Allocation /beta 1 ==
  data: u_star input; u_cmd output; alpha input; alpha_cmd output
function [ u_cmd , alpha_cmd ] = beta ( u_star , alpha )

for i=1:2
    if u_star(i) < 0
        u_star(i) = abs(u_star(i));
        alpha(i) = alpha(i) - pi;
        if alpha(i) <= -pi
            alpha(i) = alpha(i) + 2*pi ;
        end
    end
    
    if u_star(i) > 1 
        u_star(i) = 1;
    end
end

u_cmd = u_star;
alpha_cmd = alpha;

end

== matlab function Sim_3_observer_performance_no_noise/Controller/DP_Ctrl/Thrust Allocation /fixed azimuth thrust allocation  ==
  data: tau_ref input; u_cmd output; alpha input; alpha_cmd output
function [ u_cmd , alpha_cmd ] = fcn(tau_ref , alpha)

k1 = 1.030; k2 = 1.030; k3 = 2.629;
k = [k1;k2;k3];
K = diag(k);    %Thrust coefficient matrix

Lx = -0.4574; Ly = 0.055; L_BT = 0.3875;  %Thruster cooridinates

B_alpha = [                      cos(alpha(1))                     ,                   cos(alpha(2))                        ,   0 ; 
                                         sin(alpha(1))                     ,                    sin(alpha(2))                         ,   1 ;
                     - Ly * cos(alpha(1)) + Lx * sin(alpha(1)) , Ly * cos(alpha(2)) + Lx * sin(alpha(2)) , L_BT ];

u_cmd = pinv(B_alpha*K) * tau_ref;
alpha_cmd = alpha;

end

== matlab function Sim_3_observer_performance_no_noise/Controller/DP_Ctrl/Thrust Allocation /varying azimuth thrust allocation ==
  data: tau_ref input; u_cmd output; alpha_cmd output
function [ u_cmd , alpha_cmd ] = fcn(tau_ref)

k1 = 1.030; k2 = 1.030; k3 = 2.629;
k = [k1;k1;k2;k2;k3];
K = diag(k);    %Thrust coefficient matrix

Lx = -0.4574; Ly = 0.055; L_BT = 0.3875;  %Thruster cooridinates

B_alpha = [ 1, 0, 1, 0, 0 ;
            0, 1, 0, 1, 1 ;
            Ly, Lx, -Ly, Lx, L_BT];
            
u_star = pinv( B_alpha * K ) * tau_ref ;

u_cmd = zeros(3,1);
alpha_cmd = zeros(2,1);

u_cmd(1) = sqrt(u_star(1)^2 + u_star(2)^2) ;
u_cmd(2) = sqrt(u_star(3)^2 + u_star(4)^2) ;
u_cmd(3) = u_star(5) ;

alpha_cmd(1) = atan2(u_star(2),u_star(1));
alpha_cmd(2) = atan2(u_star(2),u_star(1));
end

== matlab function Sim_3_observer_performance_no_noise/Signal failure simulation, Dead reckoning function and Nonlinear Observer/WrapPsiTo[-pi,pi]2/Wrap2psi1 ==
  data: u input; yQualisus output
function yQualisus = fcn(u)
y=sin(u);
x=cos(u);
yQualisus=atan2(y,x);
end

== matlab function Sim_3_observer_performance_no_noise/Signal failure simulation, Dead reckoning function and Nonlinear Observer/WrapPsiTo[-pi,pi]1/Wrap2psi1 ==
  data: u input; yQualisus output
function yQualisus = fcn(u)
y=sin(u);
x=cos(u);
yQualisus=atan2(y,x);
end

== matlab function Sim_3_observer_performance_no_noise/Controller/CtrlCustom_SLX/Pose/Wrap2psi ==
  data: u input; yQualisus output
function yQualisus = fcn(u)
y=sin(u);
x=cos(u);
yQualisus=atan2(y,x);
end

== matlab function Sim_3_observer_performance_no_noise/Signal failure simulation, Dead reckoning function and Nonlinear Observer/Check_heading ==
  data: eta input; eta_out output
function eta_out = fcn(eta)
if(abs(eta(3,1)) > 0.5*pi && eta(3,1) < 0)
    eta(3,1) = eta(3,1) + 2*pi;
end
    eta_out = eta;

end

== matlab function Sim_3_observer_performance_no_noise/Controller/CtrlCustom_SLX/Pose/MATLAB Function ==
  data: psi input; psi_out output; psi_old input
function psi_out = fcn(psi,psi_old)
psi_out=psi_old+angdiff(psi_old,psi);

== matlab function Sim_3_observer_performance_no_noise/Controller/CtrlCustom_SLX/Backstepping controller/Backstepper controller/Backstepping controller with integral effect  ==
  data: tau_ref output size=3; pathparameter input; path_planner_data input; s_dot output size=1; eta input; nu_hat input; psi_ref input; s input; epsilon input; epsilon_dot output; Controller_Data parameter; eta_d output
function [tau_ref, s_dot, epsilon_dot,eta_d]  = fcn(pathparameter, path_planner_data, eta, nu_hat, psi_ref, s, epsilon, Controller_Data)
    %Calculation of of the different factors from manyfactors function

%Declaring constants from workspace and dealing them from Controller_Data
%from init
persistent K_p K_v K_i M D U_ref mu

    [K_p, K_v, K_i, M, D, U_ref, mu] = deal(Controller_Data.K_p,...
        Controller_Data.K_v, Controller_Data.K_i, Controller_Data.M,...
        Controller_Data.D, Controller_Data.U_ref, Controller_Data.mu);

%     K_p = Controller_Data(1:3,1:3);
%     K_v = Controller_Data(1:3,4:6);
%     K_i = Controller_Data(1:3,7:9);
%     M = Controller_Data(1:3,10:12);
%     D = Controller_Data(1:3,13:15);

    start_pos = path_planner_data(1:3); 
    end_pos = path_planner_data(4:6);
    Radius = path_planner_data (7:8);
    Center = path_planner_data(9:10);

    rx = Radius(1);
    ry = Radius(2);

    Cx = Center(1); %center of elipsoid
    Cy = Center(2);  
% 
%     Cx = (end_pos(1)-start_pos(1))/2;
%     Cy = (end_pos(2)-start_pos(2))/2;
%     rx = sqrt(Cx^2 + Cy^2);
%     ry = 1/4 * rx;

%Check if heading is close to pi/-pi and change the definition to [0,2pi];
if (abs(eta(3,1)) > 0.5*pi && eta(3,1) < 0)
    eta(3,1) = eta(3,1)+2*pi;
end

    psi_meas = eta(3,1);
%     psi = psi_ref;
    r = nu_hat(3,1);
%     integral_effect = [0; 0; yaw_V_err_integral];

%% Path planner
    if not(pathparameter) %If elipsoid
%% Calculating terms for eta and its derivatives 
        xdf = (-rx*2*pi*sin(2*pi*s)); %x_d'
        ydf = (ry*2*pi*cos(2*pi*s)); %y_d'
        xdff = -rx*(2*pi)^2*cos(2*pi*s); %x_d''
        ydff = -ry*(2*pi)^2*sin(2*pi*s); %y_d''
        xdfff = rx*(2*pi)^3*sin(2*pi*s); %x_d'''
        ydfff = -ry*(2*pi)^3*cos(2*pi*s); %y_d'''

        df_dydf =  xdf/(ydf^2+xdf^2); %df/dx_d'
        df_dxdf = -ydf/(ydf^2+xdf^2); %df/dy_d'
        ddf_dxddf = 2*xdf*ydf/(xdf^2+ydf^2)^2; %d^2f/dx_d'^2
        ddf_ddydf = -2*xdf*ydf/(xdf^2+ydf^2)^2; %d^2f/dy_d'^2
        ddf_dxdfdydf = (ydf^2-xdf^2)/(ydf^2+xdf^2)^2; %d^2f/(dx_d'dy_d')

        dh_dxdf = -U_ref*xdf/(xdf^2+ydf^2)^(3/2);
        dh_dydf = -U_ref*ydf/(xdf^2+ydf^2)^(3/2);
        
        
%% ssa 
        DesiredHeading = atan2(ydf,xdf);
        val_1 = DesiredHeading;
        val_2 = DesiredHeading + 2*pi;
        val_3 = DesiredHeading - 2*pi;

        vals = [val_1, val_2, val_3];

        [m, i] = min(abs(vals - psi_meas));

        DesiredHeading_ssa = vals(i);
%       DesiredHeading_ssa

%% Declaring the outputs
         %eta_d
%         eta_d = [Cx+rx*cos(2*pi*s), Cy+ry*sin(2*pi*s), DesiredHeading]';
        eta_d = [Cx+rx*cos(2*pi*s), Cy+ry*sin(2*pi*s), DesiredHeading_ssa]';
%         eta_d = [Cx+rx*cos(2*pi*s), Cy+ry*sin(2*pi*s), atan2(ydf,xdf)]';
        
        %eta_d'
        eta_df = [xdf, ydf, df_dxdf*xdff+df_dydf*ydff]';
        
        %eta_d''
        eta_dff = [xdff, ydff, ddf_dxddf*xdff^2+ddf_ddydf*ydff^2+2*ddf_dxdfdydf*xdff*ydff+df_dxdf*xdfff+df_dydf*ydfff]';

        %U_s'
        U_sf = dh_dxdf*xdff + dh_dydf*ydff;

        %U_s
        U_s = U_ref/sqrt(xdf^2+ydf^2);

    else %else straight line
        
        Trajectory = (end_pos(:,1) - start_pos(:,1))*s + start_pos(:,1);
%         DesiredHeading_ssa = psi_ref;

            DesiredHeading = atan2((end_pos(2,:)-start_pos(2,:)),(end_pos(1,:)-start_pos(1,:)));


%         DesiredHeading = atan((end_pos(2,:)-start_pos(2,:))/(end_pos(1,:)-start_pos(1,:)));
        
        
%         DesiredHeading
%% ssa 
        val_1 = DesiredHeading;
        val_2 = DesiredHeading + 2*pi;
        val_3 = DesiredHeading - 2*pi;

        vals = [val_1, val_2, val_3];

        [m, i] = min(abs(vals - psi_meas));

        DesiredHeading_ssa = vals(i);
%         psi_meas

        %%
        
        %eta_d
%         eta_d = transpose([Trajectory(1), Trajectory(2), DesiredHeading]);
        eta_d = transpose([Trajectory(1), Trajectory(2), DesiredHeading_ssa]);
%       eta_d = transpose([s*x2+(1-s)*x1, s*y2+(1-s)*y1, atan2(y2-y1,x2-x1)]);
        
        %eta_d'
        eta_df = transpose([end_pos(1,:) - start_pos(1,:), end_pos(2,:) - start_pos(1,:), 0]);
%       eta_df = transpose([x2-x1, y2-y1, 0]);
        
        %eta_d''
        eta_dff = transpose([0 0 0]);
        
        %U_s'
        U_sf = 0;

        %U_s
        U_s = U_ref/norm(eta_df,2);
%         U_s = U_ref/sqrt((end_pos(1,:) - start_pos(1,:))^2 + (end_pos(2,:) - start_pos(1,:))^2);
%         U_s = U_ref/sqrt((x2-x1)^2+(y2-y1)^2);
    end

%% Output calculations
    V1s = -transpose(eta-eta_d)*eta_df; %eq (38)
    
    R_psi = [ cos(psi_meas)  -sin(psi_meas)   0  ;
                    sin(psi_meas)    cos(psi_meas)  0  ; 
                        0              0         1  ] ;
    R_tr = transpose(R_psi);

    S_r = [ 0  -r   0  ;
             r  0   0   ; 
             0  0  0   ] ;   

    S_tr = transpose(S_r);

    %S_dot
    s_dot = U_s - mu*V1s/norm(eta_df,2);
    % s_dot = U_s + mu*eta_df'/norm(eta_df,2)*(eta - eta_d); %eq: 55

    %Calculate Z1_dot
    z1_dot = -S_r*R_tr*(eta - eta_d) + nu_hat - R_tr*eta_df*s_dot;

    z_1 = R_tr*(eta-eta_d);
    
    
    %Calculate d_dt
    d_dt = S_tr*R_tr*eta_df*U_s + R_tr*s_dot*(eta_dff*U_s + eta_df*U_sf);

    alpha_1_dot = -K_p*z1_dot + d_dt;
    
    alpha_1 = -K_p*z_1 + R_tr*eta_df*U_s;

    % Tau
    z_2 = nu_hat - alpha_1;
    
    %Augmenting the state space with error dynamics. Should this be z1
    %instead?
    epsilon_dot = z_2;
%     epsilon_dot = z_1;
    
%With integral effect added
%     tau_ref = D*alpha_1 + M*alpha_1_dot - K_v*z_2 + K_i*epsilon;
    tau_ref = D*alpha_1 + M*alpha_1_dot - K_v*z_2 - K_i*epsilon;
    
%Withhout integral effect
%  tau_ref = D*alpha_1 + M*alpha_1_dot - K_v*z_2;

    
end

== matlab function Sim_3_observer_performance_no_noise/Controller/CtrlCustom_SLX/Backstepping controller/MATLAB Function ==
  data: eta input; path_planner_data output; tau_select output; clock_signal input; path_planner_data_in input; tau_select_in input; tau_ref output; start_pos input
function [path_planner_data, tau_select,tau_ref] = fcn(eta,clock_signal,path_planner_data_in,tau_select_in,start_pos)
%Straight-line
% start_pos = [0;0;0];
end_pos = [10;10;0];

%Elliptical
rx = 10;
ry = 20;
Cx = 0; %center of elipsoid
Cy = 0;

path_planner_data = [start_pos ; end_pos ; rx ; ry ; Cx ; Cy];
% path_planner_data = zeros(10,1);
tau_ref = [0.1;0.1;0.1];
tau_select = tau_select_in;
if clock_signal==50
    start_pos = [eta(1);eta(2);eta(3)];
    end_pos = [cos(eta(3))*200;sin(eta(3))*200;eta(3)]
    Cx = eta(1)-rx;
    Cy = eta(2);
    path_planner_data = [start_pos ; end_pos ; rx ; ry ; Cx ; Cy];
    tau_select = 1;
end

if clock_signal > 50
    path_planner_data = path_planner_data_in;
    

end

end

== matlab function Sim_3_observer_performance_no_noise/Signal failure simulation, Dead reckoning function and Nonlinear Observer/MATLAB Function1 ==
  settings: updateMethod=DISCRETE
  data: eta input size=3; eta_out output size=3; deadreckoning output; prev_eta input; LoS_check input; stored_eta output
function [eta_out, deadreckoning, stored_eta] = Deadreck(eta, prev_eta,  LoS_check)

    if not(LoS_check) %If loss of signal is true, i.e LoS_check = 0
        dead_signal = true;
        for i = 1:3 %Check if current measurement and 3 prior positions are equal
            if eta ~= prev_eta(i,:)'
              dead_signal = false;
            end
        end
          
        if dead_signal %If four last signal values are equal, set output to be equal to eta_hat when we last had 
            deadreckoning = 1;
            eta_out = eta;

        else %Signal is not dead or frozen - Do normal stuff
            deadreckoning = 1;
            eta_out = eta;

        end
    else %If measurements are available - Do normal stuff
        deadreckoning = 0;
        eta_out = eta;
    end

stored_eta = prev_eta;
stored_eta(1:2,:) = prev_eta(end-1:end,:);
stored_eta(end,:) = eta';
end

== matlab function Sim_3_observer_performance_no_noise/Signal failure simulation, Dead reckoning function and Nonlinear Observer/Nonlinear Observer ==
  settings: updateMethod=DISCRETE
  data: eta input; eta_hat input; nu_hat input; b_hat input; eta_hat_dot output size=3; DR input; tau input; nu_hat_dot output size=3; Observergains parameter; Controller_Data parameter; b_hat_dot output size=3; eta_tilde output
function [eta_hat_dot, nu_hat_dot, b_hat_dot, eta_tilde] = Nonlinear_Observer(eta, eta_hat, nu_hat, b_hat,DR, tau, Observergains, Controller_Data)

persistent M D
    [M, D] = deal(Controller_Data.M, Controller_Data.D);

scaling = 0.01/0.1;
L1 = scaling*Observergains(1:3,1:3);
L2 = scaling*Observergains(1:3,4:6);
L3 = scaling*Observergains(1:3,7:9);

psi = eta(3,1);

R_psi = [ cos(psi)  -sin(psi)   0  ;
          sin(psi)    cos(psi)  0  ; 
          0              0         1  ] ;
R_tr = transpose(R_psi);

if DR
    L1 = 0*L1;
    L2 = 0*L2;
    L3 = 0*L3;
end
eta_tilde = eta - eta_hat;
eta_hat_dot = R_psi*nu_hat + L1*eta_tilde;
nu_hat_dot = M\(-D*nu_hat + R_tr*b_hat + tau + R_tr*L2*eta_tilde);
b_hat_dot = L3*eta_tilde;

end

== matlab function Sim_3_observer_performance_no_noise/Wrap2QualisysOutput 1/Wrap2psi ==
  data: u input; yQualisus output
function yQualisus = fcn(u)
y=sin(u);
x=cos(u);
yQualisus=atan2(y,x);
end

== matlab function Sim_3_observer_performance_no_noise/Signal failure simulation, Dead reckoning function and Nonlinear Observer/Pose1/MATLAB Function ==
  data: psi input; psi_out output; psi_old input
function psi_out = fcn(psi,psi_old)
psi_out=psi_old+angdiff(psi_old,psi);
